simulink model "teleop_sim_angle"  (R2020a)
settings: Solver=VariableStepAuto  StartTime=0.0  StopTime=20  MaxStep=dt  RelTol=1e-3
model workspace (MATLAB code in the model file):
  | run workspace_setup_scripts/teleop_sim_setup;
undefined symbols (not defined in the file): A_v, b, d_T, derivative_phases, epsilon, f_0, K_d, K_p, m, v_0, w_v, x_0
settings Model: Creator=Shane  LastModifiedBy=shfor
settings DataIOCC: ReturnWorkspaceOutputs=off
settings DebuggingCC: PregeneratedLibrarySubsystemCodeDiagnostic=none  StrictBusMsg=WarnOnBusTreatedAsVector  ArithmeticOperatorsInVariantConditions=warning
settings SFSimCC: SimUseLocalCustomCode=off  CustomCodeUndefinedFunction=UseInterfaceOnly
settings RTWCC: RTWUseLocalCustomCode=off

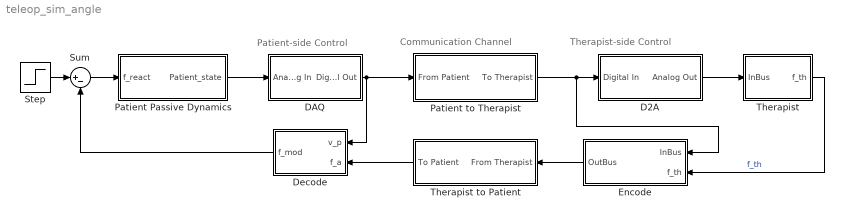
== system teleop_sim_angle ==
  note: Patient-side Control
  note: Therapist-side Control
  note: Communication Channel
  D2A : Subsystem
  DAQ : Subsystem
  Decode : Subsystem
  Encode : Subsystem
  Patient Passive Dynamics : Subsystem
  Patient to Therapist : Subsystem
  Step : Step  After=0  SampleTime=0
  Sum : Sum  Inputs=|+-
  Therapist : Subsystem
  Therapist to Patient : Subsystem
  wires:
  Sum/1 -> Patient Passive Dynamics/1(f_react)
  Patient Passive Dynamics/1(Patient_state) -> DAQ/1(Analog In)
  Step/1 -> Sum/1
  Therapist/1(f_th) -> Encode/2(f_th)  "f_th"
  Patient to Therapist/1(To Therapist) -> D2A/1(Digital In), Encode/1(InBus)
  Encode/1(OutBus) -> Therapist to Patient/1(From Therapist)
  Therapist to Patient/1(To Patient) -> Decode/2(f_a)
  Decode/1(f_mod) -> Sum/2
  DAQ/1(Digital Out) -> Decode/1(v_p), Patient to Therapist/1(From Patient)
  D2A/1(Analog Out) -> Therapist/1(InBus)

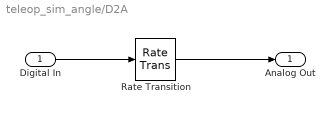
== system teleop_sim_angle/D2A ==
  Digital In : Inport
  Rate Transition : RateTransition
  Analog Out : Outport  VectorParamsAs1DForOutWhenUnconnected=off
  wires:
  Digital In/1 -> Rate Transition/1
  Rate Transition/1 -> Analog Out/1

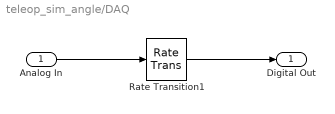
== system teleop_sim_angle/DAQ ==
  Analog In : Inport
  Rate Transition1 : RateTransition  OutPortSampleTime=Ts
  Digital Out : Outport  VectorParamsAs1DForOutWhenUnconnected=off
  wires:
  Analog In/1 -> Rate Transition1/1
  Rate Transition1/1 -> Digital Out/1

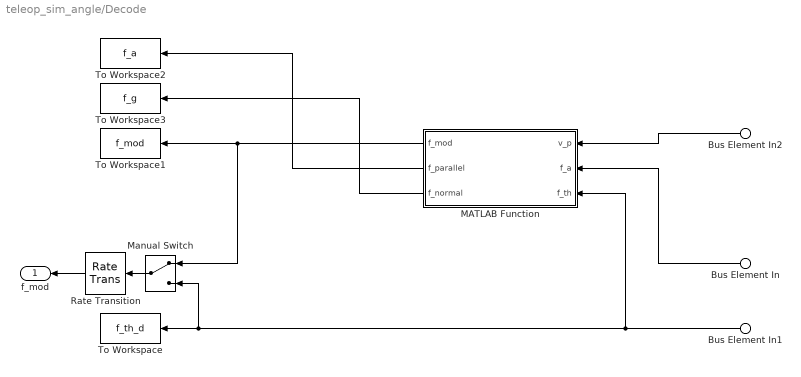
== system teleop_sim_angle/Decode ==
  Bus Element In2 : Inport  PortName=v_p  Element=v_p
  Bus Element In : Inport  Port=2  PortName=f_a  Element=f_a
  Bus Element In1 : Inport  Port=2  PortName=f_a  Element=f_th
  MATLAB Function : MATLAB Function  TreatAsAtomicUnit=on
  Manual Switch : ManualSwitch
  Rate Transition : RateTransition
  To Workspace : ToWorkspace  VariableName=f_th_d  SaveFormat=Timeseries  SampleTime=-1
  To Workspace1 : ToWorkspace  VariableName=f_mod  SaveFormat=Timeseries  SampleTime=-1
  To Workspace2 : ToWorkspace  VariableName=f_a  SaveFormat=Timeseries  SampleTime=-1
  To Workspace3 : ToWorkspace  VariableName=f_g  SaveFormat=Timeseries  SampleTime=-1
  f_mod : Outport  VectorParamsAs1DForOutWhenUnconnected=off
  wires:
  Bus Element In2/1 -> MATLAB Function/1(v_p)
  Manual Switch/1 -> Rate Transition/1
  Bus Element In1/1 -> MATLAB Function/3(f_th), Manual Switch/2, To Workspace/1
  Rate Transition/1 -> f_mod/1
  Bus Element In/1 -> MATLAB Function/2(f_a)
  MATLAB Function/1(f_mod) -> Manual Switch/1, To Workspace1/1
  MATLAB Function/2(f_parallel) -> To Workspace2/1
  MATLAB Function/3(f_normal) -> To Workspace3/1

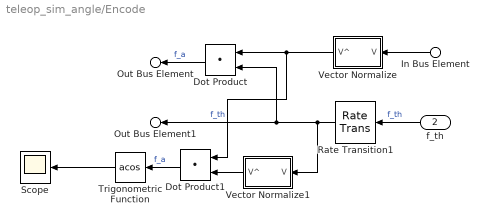
== system teleop_sim_angle/Encode ==
  In Bus Element : Inport  PortName=InBus  Element=v_p
  f_th : Inport  Port=2
  Dot Product : DotProduct  InputSameDT=on  OutDataTypeStr=Inherit: Inherit via internal rule
  Dot Product1 : DotProduct  InputSameDT=on  OutDataTypeStr=Inherit: Inherit via internal rule
  Rate Transition1 : RateTransition  InitialCondition=f_0  OutPortSampleTime=Ts
  Scope : Scope
  Trigonometric Function : Trigonometry  Operator=acos
  Vector Normalize : Subsystem  mask{min_magnitude=epsilon}
      mask prompts: min_magnitude "Minimum magnitude:"
  Vector Normalize1 : Subsystem  mask{min_magnitude=epsilon}
      mask prompts: min_magnitude "Minimum magnitude:"
  Out Bus Element : Outport  VectorParamsAs1DForOutWhenUnconnected=off  PortName=OutBus  Element=f_a
  Out Bus Element1 : Outport  VectorParamsAs1DForOutWhenUnconnected=off  PortName=OutBus  Element=f_th
  wires:
  f_th/1 -> Rate Transition1/1  "f_th"
  Dot Product/1 -> Out Bus Element/1  "f_a"
  In Bus Element/1 -> Vector Normalize/1(V)
  Rate Transition1/1 -> Vector Normalize1/1(V), Dot Product/2, Out Bus Element1/1  "f_th"
  Vector Normalize/1(V^) -> Dot Product1/1, Dot Product/1
  Vector Normalize1/1(V^) -> Dot Product1/2
  Dot Product1/1 -> Trigonometric Function/1  "f_a"
  Trigonometric Function/1 -> Scope/1

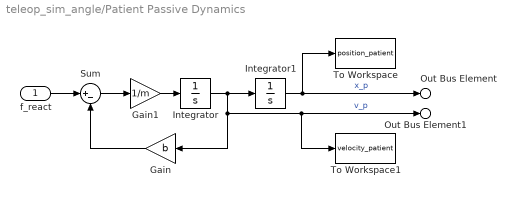
== system teleop_sim_angle/Patient Passive Dynamics ==
  f_react : Inport
  Gain : Gain  Gain=b
  Gain1 : Gain  Gain=1/m
  Integrator : Integrator  InitialCondition=v_0
  Integrator1 : Integrator  InitialCondition=x_0
  Sum : Sum  Inputs=|+-
  To Workspace : ToWorkspace  VariableName=position_patient  SaveFormat=Timeseries  SampleTime=-1
  To Workspace1 : ToWorkspace  VariableName=velocity_patient  SaveFormat=Timeseries  SampleTime=-1
  Out Bus Element : Outport  VectorParamsAs1DForOutWhenUnconnected=off  PortName=Patient_state  Element=x_p
  Out Bus Element1 : Outport  VectorParamsAs1DForOutWhenUnconnected=off  PortName=Patient_state  Element=v_p
  wires:
  Integrator/1 -> Gain/1, Out Bus Element1/1, To Workspace1/1, Integrator1/1  "v_p"
  Integrator1/1 -> To Workspace/1, Out Bus Element/1  "x_p"
  f_react/1 -> Sum/1
  Sum/1 -> Gain1/1
  Gain/1 -> Sum/2
  Gain1/1 -> Integrator/1

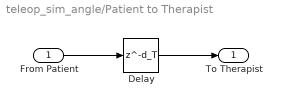
== system teleop_sim_angle/Patient to Therapist ==
  From Patient : Inport
  Delay : Delay  DelayLength=d_T
  To Therapist : Outport  VectorParamsAs1DForOutWhenUnconnected=off
  wires:
  From Patient/1 -> Delay/1
  Delay/1 -> To Therapist/1

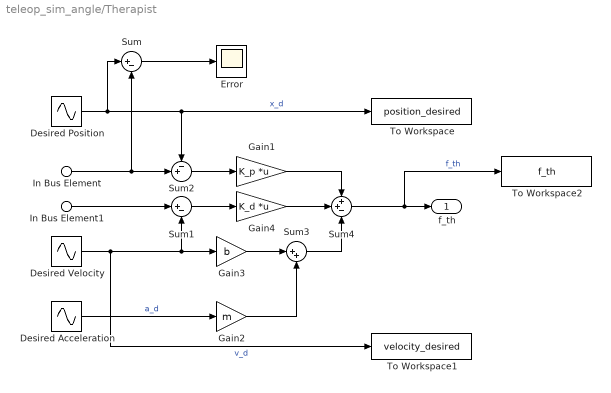
== system teleop_sim_angle/Therapist ==
  In Bus Element1 : Inport  PortName=InBus  Element=v_p
  In Bus Element : Inport  PortName=InBus  Element=x_p
  Desired Acceleration : Sin  Amplitude=-A_v*w_v^2  Frequency=w_v  Phase=derivative_phases(:,3)  SampleTime=0
  Desired Position : Sin  Amplitude=A_v  Frequency=w_v  Phase=derivative_phases(:,1)  SampleTime=0
  Desired Velocity : Sin  Amplitude=A_v*w_v  Frequency=w_v  Phase=derivative_phases(:,2)  SampleTime=0
  Error : Scope
  Gain1 : Gain  Gain=K_p  Multiplication=Matrix(K*u)
  Gain2 : Gain  Gain=m
  Gain3 : Gain  Gain=b
  Gain4 : Gain  Gain=K_d  Multiplication=Matrix(K*u)
  Sum : Sum  Inputs=|+-
  Sum1 : Sum  Inputs=|+-
  Sum2 : Sum  Inputs=-+|
  Sum3 : Sum  Inputs=|++
  Sum4 : Sum  Inputs=++-
  To Workspace : ToWorkspace  VariableName=position_desired  SaveFormat=Timeseries  SampleTime=-1
  To Workspace1 : ToWorkspace  VariableName=velocity_desired  SaveFormat=Timeseries  SampleTime=-1
  To Workspace2 : ToWorkspace  VariableName=f_th  SaveFormat=Timeseries  SampleTime=-1
  f_th : Outport  VectorParamsAs1DForOutWhenUnconnected=off
  wires:
  Desired Position/1 -> Sum/1, Sum2/1, To Workspace/1  "x_d"
  Desired Velocity/1 -> Sum1/2, Gain3/1, To Workspace1/1  "v_d"
  Sum2/1 -> Gain1/1
  Desired Acceleration/1 -> Gain2/1  "a_d"
  Gain3/1 -> Sum3/1
  Gain2/1 -> Sum3/2
  Gain1/1 -> Sum4/1
  Sum4/1 -> To Workspace2/1, f_th/1  "f_th"
  In Bus Element/1 -> Sum/2, Sum2/2
  In Bus Element1/1 -> Sum1/1
  Sum1/1 -> Gain4/1
  Sum3/1 -> Sum4/3
  Gain4/1 -> Sum4/2
  Sum/1 -> Error/1

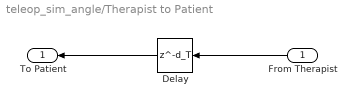
== system teleop_sim_angle/Therapist to Patient ==
  From Therapist : Inport
  Delay : Delay  DelayLength=d_T
  To Patient : Outport  VectorParamsAs1DForOutWhenUnconnected=off
  wires:
  From Therapist/1 -> Delay/1
  Delay/1 -> To Patient/1

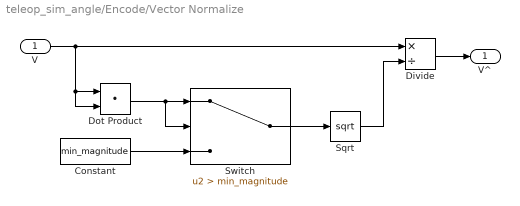
== system teleop_sim_angle/Encode/Vector Normalize ==
  V : Inport
  Constant : Constant  Value=min_magnitude
  Divide : Product  Inputs=*/
  Dot Product : DotProduct  OutMin=epsilon  InputSameDT=on  OutDataTypeStr=Inherit: Inherit via internal rule
  Sqrt : Sqrt  SaturateOnIntegerOverflow=on
  Switch : Switch  Criteria=u2 > Threshold  Threshold=min_magnitude
  V^ : Outport  VectorParamsAs1DForOutWhenUnconnected=off
  wires:
  V/1 -> Divide/1, Dot Product/1, Dot Product/2
  Divide/1 -> V^/1
  Dot Product/1 -> Switch/2, Switch/1
  Sqrt/1 -> Divide/2
  Switch/1 -> Sqrt/1
  Constant/1 -> Switch/3

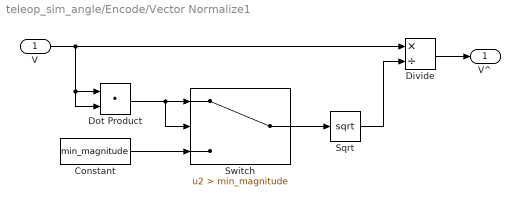
== system teleop_sim_angle/Encode/Vector Normalize1 ==
  V : Inport
  Constant : Constant  Value=min_magnitude
  Divide : Product  Inputs=*/
  Dot Product : DotProduct  OutMin=epsilon  InputSameDT=on  OutDataTypeStr=Inherit: Inherit via internal rule
  Sqrt : Sqrt  SaturateOnIntegerOverflow=on
  Switch : Switch  Criteria=u2 > Threshold  Threshold=min_magnitude
  V^ : Outport  VectorParamsAs1DForOutWhenUnconnected=off
  wires:
  Constant/1 -> Switch/3
  Switch/1 -> Sqrt/1
  Sqrt/1 -> Divide/2
  Dot Product/1 -> Switch/1, Switch/2
  Divide/1 -> V^/1
  V/1 -> Dot Product/2, Dot Product/1, Divide/1

== matlab function teleop_sim_angle/Decode/MATLAB Function ==
  data: v_p input; f_mod output; f_a input; f_th input; f_parallel output; f_normal output
function [f_mod, f_parallel, f_normal] = rotate_force(v_p, f_a, f_th)

    mag_tolerance = 1E-4;
    v_p_hat = normalize_vector(v_p, mag_tolerance);
    % Calculating the parallel component of force
    f_parallel = f_a*v_p_hat;
    % Finding the unit vector perpendicular to f_th in the direction of v_p
    n = f_th - v_p_hat*dot(v_p_hat,f_th);
    n_hat = normalize_vector(n, mag_tolerance);
    % Finding the perpendicular component of force
    f_normal = sqrt(dot(f_th,f_th) - f_a^2)*n_hat;
    
    f_mod = f_parallel + f_normal;
end

function unit_vector = normalize_vector(input_vector, tol)
    vector_mag2 = input_vector'*input_vector;
    if vector_mag2 < tol
        unit_vector = input_vector./tol;
    else
        unit_vector = input_vector./sqrt(vector_mag2);
    end
end
